simulink subsystem "rc_cmds_format"  (R2024a)
settings: Solver=VariableStepAuto  StartTime=0.0  StopTime=10.0  RelTol=1e-3
settings Model: Creator=gurt1  LastModifiedBy=gurt1

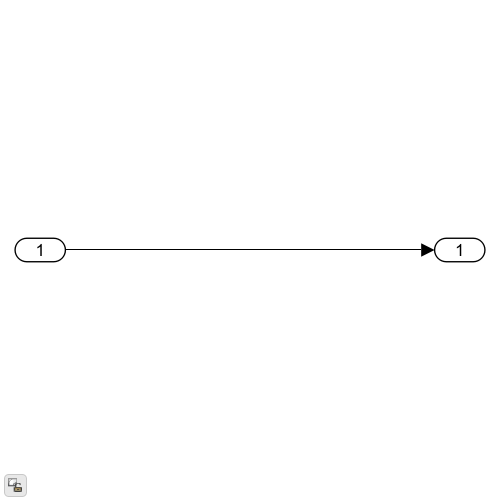
[thumbnail: Simulink's stored preview of the top-level diagram]
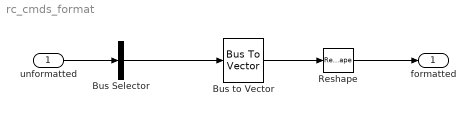
== system rc_cmds_format ==
  unformatted : Inport
  Bus Selector : BusSelector  OutputSignals=sticks,switches  OutputAsBus=on
  Bus to Vector : BusToVector
  Reshape : Reshape
  formatted : Outport
  wires:
  unformatted/1 -> Bus Selector/1
  Bus Selector/1 -> Bus to Vector/1
  Bus to Vector/1 -> Reshape/1
  Reshape/1 -> formatted/1
